simulink model "sgMdl_IO811_VideoStreamUDP"  (R2024b)
settings: Solver=FixedStepAuto  StartTime=0.0  StopTime=inf  RelTol=1e-3  EnableMultiTasking=on
model workspace (MAT data in the model file):
  Ts = 0.0333333333333
undefined symbols (not defined in the file): A1000, Aviator, Basler, FreeRun
libraries: slrealtimeutilitieslib x4, matrix_library x4, slrealtimeiplib x4, speedgoatlib_interrupt x1, speedgoatlib_IO811 x1
Description:
  | IO811 - Stream Video over UDP
settings Model: xpc_rtwmakecfg_data=_jpeg_  ModifiedByFormat=Speedgoat  SimulationMode=external  ExtModeEnableFloating=off  Creator=Speedgoat  LastModifiedBy=Speedgoat
settings SolverCC: ConcurrentTasks=on  AlgebraicLoopSolver=TrustRegion  PositivePriorityOrder=on  AutoInsertRateTranBlk=on
settings DataIOCC: SaveFormat=Array  SignalLoggingSaveFormat=ModelDataLogs  SaveOutput=off  DSMLogging=off  SaveTime=off  ReturnWorkspaceOutputs=off
settings OptimizationCC: BlockReduction=off  OptimizeBlockIOStorage=off  BufferReuse=off  ReuseModelBlockBuffer=off  GlobalBufferReuse=off  ExpressionFolding=off  ExpressionDepthLimit=2147483647  LocalBlockOutputs=off
settings DebuggingCC: UnderspecifiedInitializationDetection=Classic  MergeDetectMultiDrivingBlocksExec=none  SolverPrmCheckMsg=warning  TasksWithSamePriorityMsg=none  FcnCallInpInsideContextMsg=warning  UnconnectedInputMsg=warning  UnconnectedOutputMsg=warning  UnconnectedLineMsg=warning  StateNameClashWarn=warning  SFUnexpectedBacktrackingDiag=warning  SFNoUnconditionalDefaultTransitionDiag=warning  SFExecutionAtInitializationDiag=none  ArithmeticOperatorsInVariantConditions=warning
settings HardwareCC: ProdBitPerLong=64  ProdLongLongMode=on  ProdHWDeviceType=Intel->x86-64 (Linux 64)
settings ModelReferenceCC: EnableRefExpFcnMdlSchedulingChecks=on  PropagateSignalLabelsOutOfModel=off
settings SFSimCC: SimUseLocalCustomCode=off  CustomCodeUndefinedFunction=UseInterfaceOnly
settings RTWCC: Description=Speedgoat Real-Time Target Machine  SystemTargetFile=speedgoat.tlc  TemplateMakefile=slrealtime_default_tmf  PostCodeGenCommand=sg.model.build.makeCfg(bdroot, buildInfo);  RTWVerbose=off  RTWUseLocalCustomCode=off  Toolchain=Simulink Real-Time Toolchain  BuildConfiguration=Faster Runs  TargetLang=C++  GPUComputeCapability=3.5  DLArmComputeVersion=19.05
settings CodeAppCC: StateflowObjectComments=on
settings SimulinkRealTimeTargetCC: SubcomponentCodeInterfacePackaging=Reusable function  InstructionSetFMA=off  LogToMDFFile=off  SLRTFileLogMaxRuns=10  UseGCCFastMath=on
settings ConfigComp: CovMetricSettings=dw  CovSaveCumulativeToWorkspaceVar=on  CovSaveSingleToWorkspaceVar=on  CovExternalEMLEnable=off  CovSFcnEnable=off  CovBoundaryAbsTol=1.0e-5

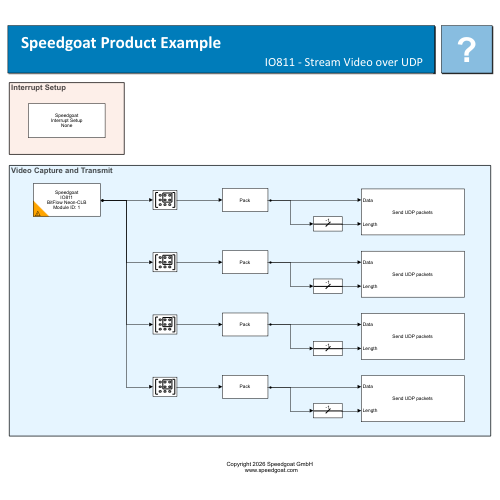
[thumbnail: Simulink's stored preview of the top-level diagram]
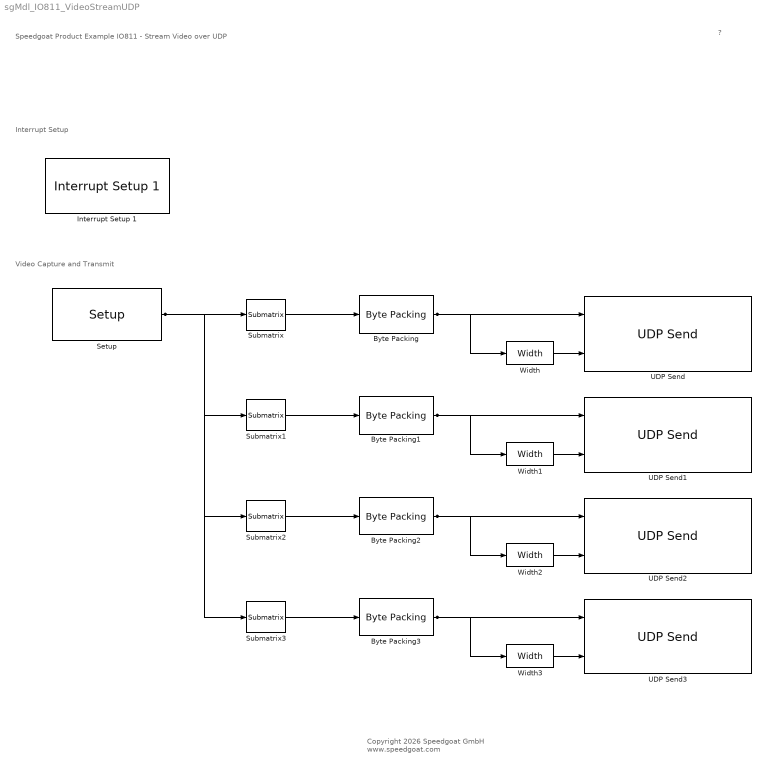
== system sgMdl_IO811_VideoStreamUDP ==
  note: Interrupt Setup
  note: Video Capture and Transmit
  note: Speedgoat Product Example
      | IO811 - Stream Video over UDP
  note: ?
  note: Copyright 2026 Speedgoat GmbH
      |  www.speedgoat.com
  Byte Packing{,1..3} (4 alike) : slrealtimeutilitieslib/Byte Packing  MaskPackedDataType=uint8  MaskUnpackedDataTypes={'uint8'}  MaskAlignment=1
  Interrupt Setup 1 : speedgoatlib_interrupt/Interrupt Setup 1  parModuleTrigger=on  parPollingMode=off  parPriorityConf=High  parPriority=254  confStartFcn=IO811_start_public  confStopFcn=IO811_stop_public  confIsrFcn=IO811_isr_public  confMapFcn=IO811_map_public  confHookFile=io811_int_hooks.c  confIrqNr=-1  confIsPolling=off  confModID=16776961  confSelectedInt=Speedgoat IO811 DMA interrupt  confSelectedId=1  confSelectedChannel=[]  confData=[]  confForcePollingMode=off
  "Setup " : speedgoatlib_IO811/Setup   camerapath=Basler-Aviator-A1000-1Kx1K-E2-FreeRun.r64  r64=CAMERA  sampletime=0.5  slot=-1  make=Basler  model=Aviator A1000  mode=8 Bits 2 Taps, 1Kx1K, Free Run  owner=BitFlow  revision=1  modelcomp=0  revcomp=0  aqtimeout=4096  format=1  flashmux=Mux_2TOEP  flashdcc=DCC  pixbitdepth=8  xsize=1024  ysize=1024  xstart=0  ystart=0  dx=500  dy=500  expmod="[1  0]"  config="[4294967295           0;4294967295          16;4294967295          16;4294967295           0;4294967295           0;4294967295           1;4294967295           0;4294967295           0;4294967295           0;4294967295           0;4294967295     4194816;4294967295           0;4294967295           0;4294967295  4294967295;4294967295         440;4294967295           0;4294967295           0;4294967295     1049088;4294967295        1024;4294967295           0;4294967295           0;4294967295   536870912;4294967295           0;4294967295           0;4294967295           0;4294967295           0;4294967295           0;4294967295           0]"  ctab="[9      0     20      1   4116      2     20      5    532      6     20     16     22     17     20  32768    256  32769      0]"  qtabmodel="[1   1024  65536]"  trigmode=0  baud=1  bytewidth=4  parity=1  stopbits=1  command="\"\""  response=0  comments=|
      | One Shot Mode
      | 
      | 
      | OVL
      | 
      | Increase Size of V0 decrease exposure.  Must also increase VReset to match.
      settings: SourceProductName=Simulink Real-Time: Speedgoat I/O Blockset
  Submatrix : matrix_library/Submatrix  RowSpan=Range of rows  RowStartMode=First  RowStartIndex=1  RowEndMode=Offset from middle  RowEndIndex=-1  ColSpan=Range of columns  ColStartMode=First  ColStartIndex=1  ColEndMode=Offset from middle  ColEndIndex=-1
  Submatrix1 : matrix_library/Submatrix  RowSpan=Range of rows  RowStartMode=Middle  RowStartIndex=1  RowEndMode=Last  RowEndIndex=1  ColSpan=Range of columns  ColStartMode=First  ColStartIndex=1  ColEndMode=Offset from middle  ColEndIndex=-1
  Submatrix2 : matrix_library/Submatrix  RowSpan=Range of rows  RowStartMode=First  RowStartIndex=1  RowEndMode=Offset from middle  RowEndIndex=-1  ColSpan=Range of columns  ColStartMode=Middle  ColStartIndex=1  ColEndMode=Last  ColEndIndex=1
  Submatrix3 : matrix_library/Submatrix  RowSpan=Range of rows  RowStartMode=Middle  RowStartIndex=1  RowEndMode=Last  RowEndIndex=1  ColSpan=Range of columns  ColStartMode=Middle  ColStartIndex=1  ColEndMode=Last  ColEndIndex=1
  UDP Send : slrealtimeiplib/UDP Send  useHostTargetConn=on  toAddress=host_ip  toPort=25000  sampleTime=-1  enableMessage=off  ipAddress=target_ip  localPort=-1
  UDP Send1 : slrealtimeiplib/UDP Send  useHostTargetConn=on  toAddress=host_ip  toPort=25001  sampleTime=-1  enableMessage=off  ipAddress=target_ip  localPort=-1
  UDP Send2 : slrealtimeiplib/UDP Send  useHostTargetConn=on  toAddress=host_ip  toPort=25002  sampleTime=-1  enableMessage=off  ipAddress=target_ip  localPort=-1
  UDP Send3 : slrealtimeiplib/UDP Send  useHostTargetConn=on  toAddress=host_ip  toPort=25003  sampleTime=-1  enableMessage=off  ipAddress=target_ip  localPort=-1
  Width{,1..3} (4 alike) : Width
  wires:
  Byte Packing/1 -> UDP Send/1, Width/1
  Width/1 -> UDP Send/2
  "Setup "/1 -> Submatrix3/1, Submatrix2/1, Submatrix1/1, Submatrix/1
  Submatrix/1 -> Byte Packing/1
  Submatrix1/1 -> Byte Packing1/1
  Width1/1 -> UDP Send1/2
  Byte Packing1/1 -> Width1/1, UDP Send1/1
  Byte Packing3/1 -> UDP Send3/1, Width3/1
  Width3/1 -> UDP Send3/2
  Submatrix3/1 -> Byte Packing3/1
  Submatrix2/1 -> Byte Packing2/1
  Width2/1 -> UDP Send2/2
  Byte Packing2/1 -> Width2/1, UDP Send2/1
